simulink model "Todo_EKF_1er_Riccati"  (R2018b)
settings: Solver=FixedStepDiscrete  StartTime=0.0  StopTime=60  FixedStep=0.02  RelTol=1e-3  EnableMultiTasking=on
InitFcn:
  | load('Pose_integration_R_L.mat')
  | ProcNoiseD=0.01^2; % is a variance
  | ProcNoiseTheta=0.001^2; % is a variance
StopFcn:
  | I = imread('Enviroment.png');
  | x = [0 35.9];
  | y=[23.31 0];
  | image(I,'XData',x,'YData',y);
  | axis xy;
  | hold on
  | .....
  | .....
  | len=length(Pose_t......);
  | for i=1:round(len/15):len
  |     plot_ellipse(Pk.signals.values(1:2,1:2,i),[xEst.signals.values(i,1), xEst.signals.values(i,2)],'g');
  | end
settings Model: Creator=antonio  LastModifiedBy=pujazon
settings DataIOCC: LimitDataPoints=on  SaveFormat=Array
settings OptimizationCC: LifeSpan=inf
settings DebuggingCC: UnderspecifiedInitializationDetection=Classic  MergeDetectMultiDrivingBlocksExec=none  SolverPrmCheckMsg=warning  StateNameClashWarn=warning  SFUnexpectedBacktrackingDiag=warning  SFNoUnconditionalDefaultTransitionDiag=warning  SFExecutionAtInitializationDiag=none
settings HardwareCC: ProdBitPerPointer=32  ProdBitPerSizeT=32  ProdBitPerPtrDiffT=32  ProdLargestAtomicFloat=None  ProdIntDivRoundTo=Undefined  ProdEndianess=Unspecified  ProdWordSize=32  ProdHWDeviceType=32-bit Generic
settings ModelReferenceCC: PropagateSignalLabelsOutOfModel=off
settings SFSimCC: SimUseLocalCustomCode=off
settings RTWCC: RTWUseLocalCustomCode=off
settings CodeAppCC: StateflowObjectComments=on
settings GRTTargetCC: TargetLangStandard=C89/C90 (ANSI)  GeneratePreprocessorConditionals=Disable all
settings ConfigComp: CovMetricSettings=dw  CovHtmlReporting=on  CovSaveCumulativeToWorkspaceVar=on  CovSaveSingleToWorkspaceVar=on  CovExternalEMLEnable=off

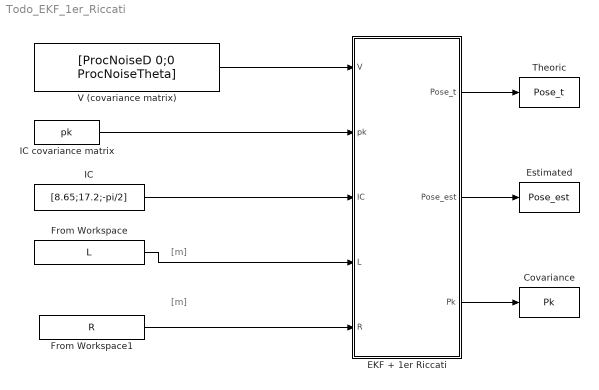
== system Todo_EKF_1er_Riccati ==
  note: [m]
  note: [m]
  Covariance : ToWorkspace  VariableName=Pk  SaveFormat=Structure With Time  SampleTime=-1
  EKF + 1er Riccati : MATLAB Function  TreatAsAtomicUnit=on
  Estimated : ToWorkspace  VariableName=Pose_est  SaveFormat=Timeseries  SampleTime=-1
  From Workspace : FromWorkspace  VariableName=L  SampleTime=0
  From Workspace1 : FromWorkspace  VariableName=R  SampleTime=0
  IC : Constant  Value=[8.65;17.2;-pi/2]
  IC covariance matrix : FromWorkspace  VariableName=pk
  Theoric : ToWorkspace  VariableName=Pose_t  SaveFormat=Timeseries  SampleTime=-1
  V (covariance matrix) : Constant  Value=[ProcNoiseD 0;0 ProcNoiseTheta]  VectorParams1D=off
  wires:
  IC/1 -> EKF + 1er Riccati/3(IC)
  EKF + 1er Riccati/1(Pose_t) -> Theoric/1
  EKF + 1er Riccati/2(Pose_est) -> Estimated/1
  From Workspace1/1 -> EKF + 1er Riccati/5(R)
  From Workspace/1 -> EKF + 1er Riccati/4(L)
  V (covariance matrix)/1 -> EKF + 1er Riccati/1(V)
  IC covariance matrix/1 -> EKF + 1er Riccati/2(pk)
  EKF + 1er Riccati/3(Pk) -> Covariance/1

== matlab function Todo_EKF_1er_Riccati/EKF + 1er Riccati ==
  data: V input; pk input; Pose_t output; Pose_est output; IC input; L input; R input; Pk output
function [Pose_t,Pose_est,Pk] = fcn(V,pk,IC,L,R) % IC->Initial Condition [xo,yo,th0]
                                   % R and L are the displacements of
                                   % wheels [m]
persistent x_w y_w suma_theta e_x e_y e_t Pkp %  internal variable to be mantain its values

ts=0.02; % sample time
S = 4;

%%%%%%%%%%%%%%%%%%%%%%%%%%%%%%%%%%%%%%%%%%%%%%%%%%%%%%%%%%%%%%%%%%%%%%%%%%
% %%%%%%%%%%%%%%   Read Initial condition   %%%%%%%%%%%%%%%%%%%%%%%%%%%%%%
x_ini=IC(1);
y_ini=IC(2);
theta_ini=IC(3);

e_x_i=IC(1);
e_y_i=IC(2);
e_t_i=IC(3);

%%%%%%%%%%%%%%%%%%%%%%%%%%%%%%%%%%%%%%%%%%%%%%%%%%%%%%%%%%%%%%%%%%%%%%%%%%
%%%%%%%%%%%%%%%   variable initialitation  %%%%%%%%%%%%%%%%%%%%%%%%%%%%%%
if isempty (x_w)
    x_w=x_ini;
    y_w=y_ini;
    suma_theta=theta_ini;
    
    e_x=e_x_i;
    e_y=e_y_i;
    e_t=e_t_i;
    
    Pkp = pk;
    
end
%%%%%%%%%%%%%%%%%%%%%%%%%%%%%%%%%%%%%%%%%%%%%%%%%%%%%%%%%%%%%%%%%%%%%%%%%%
%%%%%%%%%%%%%%%%%  compute the odometry    %%%%%%%%%%%%%%%%%%%%%%%%%%%%%%%

delta_th= (R-L)/(2*S);
delta_d = (R+L)/2;

vd=V(1,1);
vth=V(2,2);

%%%%%%%%%%%%%%%%%%%%%%%%%%%%%%%%%%%%%%%%%%%%%%%%%%%%%%%%%%%%%%%%%%%%%%%%%%
%%%%%%%%%%%%%%%%%  integration of the robot pose %%%%%%%%%%%%%%%%%%%%%%%%%%
theta_i = suma_theta;
X=[x_w;y_w;suma_theta];
E=[e_x;e_y;e_t];

x_w= x_w + ((delta_d+vd)*sin(suma_theta+delta_th+vth));
y_w= y_w + ((delta_d+vd)*sin(suma_theta+delta_th+vth));
suma_theta=mod(suma_theta+delta_th+vth,2*pi);

%Se usaria en el jacobian
%X_1=[x_w y_w suma_theta];

%%%%%%%%%%%%%%%%%  Build the Jacocian %%%%%%%%%%%%%%%%%%%%%%%%%%%%%%%%%%%%
%Fx = jacobian([x_w y_w suma_theta],[x_w y_w suma_theta]);
%Fv = jacobian([x_w y_w suma_theta],[vd,vth]);

Fx= [1 0 -(delta_d*sin(theta_i)*delta_th);...
    0 1 (delta_d*sin(theta_i)*delta_th);...
    0 0 1 ];

Fv =[cos(theta_i+delta_th) -delta_d*sin(theta_i+delta_th);...
    sin(theta_i+delta_th) delta_d*cos(theta_i+delta_th);...
    0 1];


%%%%%%%%%%%%%%%%% Compute the EKF Trucated Taylor %%%%%%%%%%%%%%%%%%%%%%%%

E_1 = E+(Fx*(X-E))+(Fv.*V);

e_x=E_1(1);
e_y=E_1(2);
e_t=E_1(3);

Pkp = Pk0;
%%%%%%%%%%%%%%%%%%%%%%%%%%%%%%%%%%%%%%%%%%%%%%%%%%%%%%%%%%%%%%%%%%%%%%%%%%
%%%%%%%%%%%%%%%%%  output variable %%%%%%%%%%%%%%%%%%%%%%%%%%%%%%%%%%%%%%%

Pose_t = P;
Pose_est = E;
Pk = Pkp;

end
